simulink model "eovsa_corr_300mhz"  (R2012b)
settings: Solver=VariableStepDiscrete  SolverMode=SingleTasking  StartTime=0.0  StopTime=5000  RelTol=1e-3
undefined symbols (not defined in the file or in its folder): A, B, gcbh, PCIN, sfp, xlBlockLoadCallback, xlipgetpartsetting
libraries: xbsIndex_r4 x5996, casper_library_misc x52, simulink x33, dspsigops x24, xps_library x15, casper_library_delays x2
(part 4 of 65)

== system eovsa_corr_300mhz/auto_shutoff1 ==
  In1 : Inport
  In2 : Inport  Port=2
  In3 : Inport  Port=3
  In4 : Inport  Port=4
  rst : Inport  Port=5
  Accumulator : xbsIndex_r4/Accumulator  operation=Add  n_bits=ceil(log2(clk_freq*1000*acc_time))+bits_in*2  overflow=Wrap  scale=1  rst=on  infoeditControl=reset for floating point data type must be asserted for a minimum of 2 cycles  hasbypass=off  en=off  latency=0  dbl_ovrd=off  msb_inp=100  msb=100  lsb=-100  use_behavioral_HDL=off  implementation=DSP48  block_type=accum
      settings: xl_area=[0, 0, 0, 0, 0, 0, 0]  block_version=10.1.3
  Constant : xbsIndex_r4/Constant  const=2^ceil(log2(clk_freq*1000*acc_time))*max_power  gui_display_data_type=Fixed-point  arith_type=Unsigned  n_bits=ceil(log2(clk_freq*1000*acc_time))+bits_in*2  bin_pt=bin_pt_in*2  preci_type=Single  exp_width=8  frac_width=24  explicit_period=on  period=1  equ=P=C  opselect=C  inp2=PCIN>>17  opr=+  inp1=P  carry=CIN  dbl_ovrd=off  block_type=constant
      settings: block_version=11.4
  Counter1 : xbsIndex_r4/Counter  cnt_type=Free Running  cnt_to=Inf  operation=Up  start_count=0  cnt_by_val=1  arith_type=Unsigned  n_bits=ceil(log2(clk_freq*1000*acc_time))+1  bin_pt=0  load_pin=off  rst=off  en=off  explicit_period=on  period=1  dbl_ovrd=off  use_behavioral_HDL=off  implementation=DSP48  use_rpm=on  block_type=counter
      settings: xl_area=[0, 0, 0, 0, 0, 0, 0]
  Counter2 : xbsIndex_r4/Counter  cnt_type=Free Running  cnt_to=Inf  operation=Up  start_count=0  cnt_by_val=1  arith_type=Unsigned  n_bits=2  bin_pt=0  load_pin=off  rst=off  en=off  explicit_period=on  period=1  dbl_ovrd=off  use_behavioral_HDL=off  implementation=Fabric  block_type=counter
      settings: block_version=11.4
  Delay4 : xbsIndex_r4/Delay  rst=off  infoeditControl=Selection of Reset will increase slice count due to use of real FFs and instead of SRLs  en=off  latency=1  dbl_ovrd=off  reg_retiming=off  block_type=delay
      settings: block_version=11.4
  Logical : xbsIndex_r4/Logical  logical_function=OR  inputs=2  en=off  latency=1  precision=Full  arith_type=Unsigned  n_bits=16  bin_pt=0  align_bp=on  dbl_ovrd=off  block_type=logical
      settings: block_version=11.4
  Mult : xbsIndex_r4/Mult  precision=Full  arith_type="Signed  (2's comp)"  n_bits=8  bin_pt=2  quantization=Truncate  overflow=Wrap  en=off  latency=3  dbl_ovrd=off  use_behavioral_HDL=off  opt=Speed  use_embedded=on  optimum_pipeline=off  pipeline=on  use_rpm=on  placement_style=Rectangular shape  block_type=mult
      settings: xl_area=[0, 0, 0, 0, 0, 0, 0]  block_version=10.1.3
  Mux : xbsIndex_r4/Mux  inputs=4  en=off  latency=1  precision=Full  arith_type="Signed  (2's comp)"  n_bits=8  bin_pt=2  quantization=Truncate  overflow=Wrap  dbl_ovrd=off  block_type=mux
      settings: xl_area=[0, 0, 0, 0, 0, 0, 0]
  Relational : xbsIndex_r4/Relational  mode=a>b  en=off  latency=1  dbl_ovrd=off  block_type=relational
  Slice : xbsIndex_r4/Slice  nbits=1  boolean_output=off  mode=Upper Bit Location + Width  bit1=0  base1=MSB of Input  bit0=0  base0=LSB of Input  dbl_ovrd=off  block_type=slice
      settings: block_version=10.1.3
  Slice1 : xbsIndex_r4/Slice  nbits=1  boolean_output=on  mode=Upper Bit Location + Width  bit1=0  base1=MSB of Input  bit0=0  base0=LSB of Input  dbl_ovrd=off  block_type=slice
  edge_detect : Subsystem  AncestorBlock=casper_library_misc/edge_detect  mask(edge_detect){edge=Both, polarity=Active High, x_in=[0 0.08 0.08 0.16 0.16 0.24 0.24 0.32 0.32 0.4], y_in=[-1 -1  1  1  1  1 -1 -1 -1 -1], x_out=[0.6 0.68 0.68 0.76 0.76 0.84 0.84 0.92 0.92 1], y_out=[-1 -1  1  1 -1 -1  1  1 -1 -1]}
      mask prompts: edge "Edge Type"; polarity "Output Polarity"; x_in "Input X Positions"; y_in "Input Y Positions"; x_out "Output X Positions"; y_out "Output Y Positions"
      mask help: Output is active for one-cycle after each edge of the specified type (i.e. rising, falling or both).
      mask init: same as eovsa_corr_300mhz/edge_detect1
      settings: AttributesFormatString=|
      | both edges
      | active high
      mask Help: Output is active for one-cycle after each edge of the specified type (i.e. rising, falling, or both).  Latency is zero.
      mask TypeOptions edge: Rising | Falling | Both
      mask TypeOptions polarity: Active High | Active Low
      mask Display:
      | plot(x_in_num,0.5+y_in_num*0.2);
      | plot(x_out_num,0.5+y_out_num*0.2);
  en : Outport
  wires:
  Delay4/1 -> Accumulator/1
  Logical/1 -> Accumulator/2
  edge_detect/1(out) -> Slice1/1
  rst/1 -> Logical/2
  Relational/1 -> en/1
  Constant/1 -> Relational/2
  In4/1 -> Mux/5
  In2/1 -> Mux/4
  In3/1 -> Mux/3
  In1/1 -> Mux/2
  Counter2/1 -> Mux/1
  Mux/1 -> Mult/2, Mult/1
  Slice/1 -> edge_detect/1(in)
  Counter1/1 -> Slice/1
  Accumulator/1 -> Relational/1
  Mult/1 -> Delay4/1
  Slice1/1 -> Logical/1

== system eovsa_corr_300mhz/auto_shutoff2 ==
  In1 : Inport
  In2 : Inport  Port=2
  In3 : Inport  Port=3
  In4 : Inport  Port=4
  rst : Inport  Port=5
  Accumulator : xbsIndex_r4/Accumulator  operation=Add  n_bits=ceil(log2(clk_freq*1000*acc_time))+bits_in*2  overflow=Wrap  scale=1  rst=on  infoeditControl=reset for floating point data type must be asserted for a minimum of 2 cycles  hasbypass=off  en=off  latency=0  dbl_ovrd=off  msb_inp=100  msb=100  lsb=-100  use_behavioral_HDL=off  implementation=DSP48  block_type=accum
      settings: xl_area=[0, 0, 0, 0, 0, 0, 0]  block_version=10.1.3
  Constant : xbsIndex_r4/Constant  const=2^ceil(log2(clk_freq*1000*acc_time))*max_power  gui_display_data_type=Fixed-point  arith_type=Unsigned  n_bits=ceil(log2(clk_freq*1000*acc_time))+bits_in*2  bin_pt=bin_pt_in*2  preci_type=Single  exp_width=8  frac_width=24  explicit_period=on  period=1  equ=P=C  opselect=C  inp2=PCIN>>17  opr=+  inp1=P  carry=CIN  dbl_ovrd=off  block_type=constant
      settings: block_version=11.4
  Counter1 : xbsIndex_r4/Counter  cnt_type=Free Running  cnt_to=Inf  operation=Up  start_count=0  cnt_by_val=1  arith_type=Unsigned  n_bits=ceil(log2(clk_freq*1000*acc_time))+1  bin_pt=0  load_pin=off  rst=off  en=off  explicit_period=on  period=1  dbl_ovrd=off  use_behavioral_HDL=off  implementation=DSP48  use_rpm=on  block_type=counter
      settings: xl_area=[0, 0, 0, 0, 0, 0, 0]
  Counter2 : xbsIndex_r4/Counter  cnt_type=Free Running  cnt_to=Inf  operation=Up  start_count=0  cnt_by_val=1  arith_type=Unsigned  n_bits=2  bin_pt=0  load_pin=off  rst=off  en=off  explicit_period=on  period=1  dbl_ovrd=off  use_behavioral_HDL=off  implementation=Fabric  block_type=counter
      settings: block_version=11.4
  Delay4 : xbsIndex_r4/Delay  rst=off  infoeditControl=Selection of Reset will increase slice count due to use of real FFs and instead of SRLs  en=off  latency=1  dbl_ovrd=off  reg_retiming=off  block_type=delay
      settings: block_version=11.4
  Logical : xbsIndex_r4/Logical  logical_function=OR  inputs=2  en=off  latency=1  precision=Full  arith_type=Unsigned  n_bits=16  bin_pt=0  align_bp=on  dbl_ovrd=off  block_type=logical
      settings: block_version=11.4
  Mult : xbsIndex_r4/Mult  precision=Full  arith_type="Signed  (2's comp)"  n_bits=8  bin_pt=2  quantization=Truncate  overflow=Wrap  en=off  latency=3  dbl_ovrd=off  use_behavioral_HDL=off  opt=Speed  use_embedded=on  optimum_pipeline=off  pipeline=on  use_rpm=on  placement_style=Rectangular shape  block_type=mult
      settings: xl_area=[0, 0, 0, 0, 0, 0, 0]  block_version=10.1.3
  Mux : xbsIndex_r4/Mux  inputs=4  en=off  latency=1  precision=Full  arith_type="Signed  (2's comp)"  n_bits=8  bin_pt=2  quantization=Truncate  overflow=Wrap  dbl_ovrd=off  block_type=mux
      settings: xl_area=[0, 0, 0, 0, 0, 0, 0]
  Relational : xbsIndex_r4/Relational  mode=a>b  en=off  latency=1  dbl_ovrd=off  block_type=relational
  Slice : xbsIndex_r4/Slice  nbits=1  boolean_output=off  mode=Upper Bit Location + Width  bit1=0  base1=MSB of Input  bit0=0  base0=LSB of Input  dbl_ovrd=off  block_type=slice
      settings: block_version=10.1.3
  Slice1 : xbsIndex_r4/Slice  nbits=1  boolean_output=on  mode=Upper Bit Location + Width  bit1=0  base1=MSB of Input  bit0=0  base0=LSB of Input  dbl_ovrd=off  block_type=slice
  edge_detect : Subsystem  AncestorBlock=casper_library_misc/edge_detect  mask(edge_detect){edge=Both, polarity=Active High, x_in=[0 0.08 0.08 0.16 0.16 0.24 0.24 0.32 0.32 0.4], y_in=[-1 -1  1  1  1  1 -1 -1 -1 -1], x_out=[0.6 0.68 0.68 0.76 0.76 0.84 0.84 0.92 0.92 1], y_out=[-1 -1  1  1 -1 -1  1  1 -1 -1]}
      mask prompts: edge "Edge Type"; polarity "Output Polarity"; x_in "Input X Positions"; y_in "Input Y Positions"; x_out "Output X Positions"; y_out "Output Y Positions"
      mask help: Output is active for one-cycle after each edge of the specified type (i.e. rising, falling or both).
      mask init: same as eovsa_corr_300mhz/edge_detect1
      settings: AttributesFormatString=|
      | both edges
      | active high
      mask Help: Output is active for one-cycle after each edge of the specified type (i.e. rising, falling, or both).  Latency is zero.
      mask TypeOptions edge: Rising | Falling | Both
      mask TypeOptions polarity: Active High | Active Low
      mask Display:
      | plot(x_in_num,0.5+y_in_num*0.2);
      | plot(x_out_num,0.5+y_out_num*0.2);
  en : Outport
  wires:
  Slice1/1 -> Logical/1
  Mult/1 -> Delay4/1
  Accumulator/1 -> Relational/1
  Counter1/1 -> Slice/1
  Slice/1 -> edge_detect/1(in)
  Mux/1 -> Mult/1, Mult/2
  Counter2/1 -> Mux/1
  In1/1 -> Mux/2
  In3/1 -> Mux/3
  In2/1 -> Mux/4
  In4/1 -> Mux/5
  Constant/1 -> Relational/2
  Relational/1 -> en/1
  rst/1 -> Logical/2
  edge_detect/1(out) -> Slice1/1
  Logical/1 -> Accumulator/2
  Delay4/1 -> Accumulator/1

== system eovsa_corr_300mhz/auto_shutoff3 ==
  In1 : Inport
  In2 : Inport  Port=2
  In3 : Inport  Port=3
  In4 : Inport  Port=4
  rst : Inport  Port=5
  Accumulator : xbsIndex_r4/Accumulator  operation=Add  n_bits=ceil(log2(clk_freq*1000*acc_time))+bits_in*2  overflow=Wrap  scale=1  rst=on  infoeditControl=reset for floating point data type must be asserted for a minimum of 2 cycles  hasbypass=off  en=off  latency=0  dbl_ovrd=off  msb_inp=100  msb=100  lsb=-100  use_behavioral_HDL=off  implementation=DSP48  block_type=accum
      settings: xl_area=[0, 0, 0, 0, 0, 0, 0]  block_version=10.1.3
  Constant : xbsIndex_r4/Constant  const=2^ceil(log2(clk_freq*1000*acc_time))*max_power  gui_display_data_type=Fixed-point  arith_type=Unsigned  n_bits=ceil(log2(clk_freq*1000*acc_time))+bits_in*2  bin_pt=bin_pt_in*2  preci_type=Single  exp_width=8  frac_width=24  explicit_period=on  period=1  equ=P=C  opselect=C  inp2=PCIN>>17  opr=+  inp1=P  carry=CIN  dbl_ovrd=off  block_type=constant
      settings: block_version=11.4
  Counter1 : xbsIndex_r4/Counter  cnt_type=Free Running  cnt_to=Inf  operation=Up  start_count=0  cnt_by_val=1  arith_type=Unsigned  n_bits=ceil(log2(clk_freq*1000*acc_time))+1  bin_pt=0  load_pin=off  rst=off  en=off  explicit_period=on  period=1  dbl_ovrd=off  use_behavioral_HDL=off  implementation=DSP48  use_rpm=on  block_type=counter
      settings: xl_area=[0, 0, 0, 0, 0, 0, 0]
  Counter2 : xbsIndex_r4/Counter  cnt_type=Free Running  cnt_to=Inf  operation=Up  start_count=0  cnt_by_val=1  arith_type=Unsigned  n_bits=2  bin_pt=0  load_pin=off  rst=off  en=off  explicit_period=on  period=1  dbl_ovrd=off  use_behavioral_HDL=off  implementation=Fabric  block_type=counter
      settings: block_version=11.4
  Delay4 : xbsIndex_r4/Delay  rst=off  infoeditControl=Selection of Reset will increase slice count due to use of real FFs and instead of SRLs  en=off  latency=1  dbl_ovrd=off  reg_retiming=off  block_type=delay
      settings: block_version=11.4
  Logical : xbsIndex_r4/Logical  logical_function=OR  inputs=2  en=off  latency=1  precision=Full  arith_type=Unsigned  n_bits=16  bin_pt=0  align_bp=on  dbl_ovrd=off  block_type=logical
      settings: block_version=11.4
  Mult : xbsIndex_r4/Mult  precision=Full  arith_type="Signed  (2's comp)"  n_bits=8  bin_pt=2  quantization=Truncate  overflow=Wrap  en=off  latency=3  dbl_ovrd=off  use_behavioral_HDL=off  opt=Speed  use_embedded=on  optimum_pipeline=off  pipeline=on  use_rpm=on  placement_style=Rectangular shape  block_type=mult
      settings: xl_area=[0, 0, 0, 0, 0, 0, 0]  block_version=10.1.3
  Mux : xbsIndex_r4/Mux  inputs=4  en=off  latency=1  precision=Full  arith_type="Signed  (2's comp)"  n_bits=8  bin_pt=2  quantization=Truncate  overflow=Wrap  dbl_ovrd=off  block_type=mux
      settings: xl_area=[0, 0, 0, 0, 0, 0, 0]
  Relational : xbsIndex_r4/Relational  mode=a>b  en=off  latency=1  dbl_ovrd=off  block_type=relational
  Slice : xbsIndex_r4/Slice  nbits=1  boolean_output=off  mode=Upper Bit Location + Width  bit1=0  base1=MSB of Input  bit0=0  base0=LSB of Input  dbl_ovrd=off  block_type=slice
      settings: block_version=10.1.3
  Slice1 : xbsIndex_r4/Slice  nbits=1  boolean_output=on  mode=Upper Bit Location + Width  bit1=0  base1=MSB of Input  bit0=0  base0=LSB of Input  dbl_ovrd=off  block_type=slice
  edge_detect : Subsystem  AncestorBlock=casper_library_misc/edge_detect  mask(edge_detect){edge=Both, polarity=Active High, x_in=[0 0.08 0.08 0.16 0.16 0.24 0.24 0.32 0.32 0.4], y_in=[-1 -1  1  1  1  1 -1 -1 -1 -1], x_out=[0.6 0.68 0.68 0.76 0.76 0.84 0.84 0.92 0.92 1], y_out=[-1 -1  1  1 -1 -1  1  1 -1 -1]}
      mask prompts: edge "Edge Type"; polarity "Output Polarity"; x_in "Input X Positions"; y_in "Input Y Positions"; x_out "Output X Positions"; y_out "Output Y Positions"
      mask help: Output is active for one-cycle after each edge of the specified type (i.e. rising, falling or both).
      mask init: same as eovsa_corr_300mhz/edge_detect1
      settings: AttributesFormatString=|
      | both edges
      | active high
      mask Help: Output is active for one-cycle after each edge of the specified type (i.e. rising, falling, or both).  Latency is zero.
      mask TypeOptions edge: Rising | Falling | Both
      mask TypeOptions polarity: Active High | Active Low
      mask Display:
      | plot(x_in_num,0.5+y_in_num*0.2);
      | plot(x_out_num,0.5+y_out_num*0.2);
  en : Outport
  wires:
  Delay4/1 -> Accumulator/1
  Logical/1 -> Accumulator/2
  edge_detect/1(out) -> Slice1/1
  rst/1 -> Logical/2
  Relational/1 -> en/1
  Constant/1 -> Relational/2
  In4/1 -> Mux/5
  In2/1 -> Mux/4
  In3/1 -> Mux/3
  In1/1 -> Mux/2
  Counter2/1 -> Mux/1
  Mux/1 -> Mult/2, Mult/1
  Slice/1 -> edge_detect/1(in)
  Counter1/1 -> Slice/1
  Accumulator/1 -> Relational/1
  Mult/1 -> Delay4/1
  Slice1/1 -> Logical/1

== system eovsa_corr_300mhz/bus_create ==
  in1 : Inport
  in2 : Inport  Port=2
  in3 : Inport  Port=3
  in4 : Inport  Port=4
  in5 : Inport  Port=5
  in6 : Inport  Port=6
  in7 : Inport  Port=7
  in8 : Inport  Port=8
  concatenate : xbsIndex_r4/Concat  num_inputs=8  dbl_ovrd=off  block_type=concat
  reinterpret{1..8} (8 alike) : xbsIndex_r4/Reinterpret  force_arith_type=on  arith_type=Unsigned  force_bin_pt=on  bin_pt=0  block_type=reinterpret
      reinterpret1 settings: infoedit="Changes signal type without altering the binary representation.   You can changed the signal between signed and unsigned, and relocate the binary point.<br><br>Hardware notes: In hardware this block costs nothing.<br><br>Example:  Suppose the input is 6 bits wide, signed, with 2 fractional bits, and the output is forced to unsigned with 0 fractional bits.  Then an input of -2.0 (1110.00 in binary 2's complement) becomes an output of 56 (111000 in binary)."
      reinterpret2 settings: infoedit="Changes signal type without altering the binary representation.   You can changed the signal between signed and unsigned, and relocate the binary point.<br><br>Hardware notes: In hardware this block costs nothing.<br><br>Example:  Suppose the input is 6 bits wide, signed, with 2 fractional bits, and the output is forced to unsigned with 0 fractional bits.  Then an input of -2.0 (1110.00 in binary 2's complement) becomes an output of 56 (111000 in binary)."
  bus_out : Outport
  wires:
  concatenate/1 -> bus_out/1
  in1/1 -> reinterpret1/1
  reinterpret1/1 -> concatenate/1
  in2/1 -> reinterpret2/1
  reinterpret2/1 -> concatenate/2
  in3/1 -> reinterpret3/1
  reinterpret3/1 -> concatenate/3
  in4/1 -> reinterpret4/1
  reinterpret4/1 -> concatenate/4
  in5/1 -> reinterpret5/1
  reinterpret5/1 -> concatenate/5
  in6/1 -> reinterpret6/1
  reinterpret6/1 -> concatenate/6
  in7/1 -> reinterpret7/1
  reinterpret7/1 -> concatenate/7
  in8/1 -> reinterpret8/1
  reinterpret8/1 -> concatenate/8

== system eovsa_corr_300mhz/bus_expand7 ==
  bus_in : Inport
  reinterpret{1..4} (4 alike) : xbsIndex_r4/Reinterpret  force_arith_type=on  arith_type=Unsigned  force_bin_pt=on  bin_pt=0  block_type=reinterpret
  slice1 : xbsIndex_r4/Slice  nbits=32  boolean_output=off  mode=Upper Bit Location + Width  bit1=-96  base1=MSB of Input  bit0=0  base0=LSB of Input  dbl_ovrd=off  block_type=slice
  slice2 : xbsIndex_r4/Slice  nbits=32  boolean_output=off  mode=Upper Bit Location + Width  bit1=-64  base1=MSB of Input  bit0=0  base0=LSB of Input  dbl_ovrd=off  block_type=slice
  slice3 : xbsIndex_r4/Slice  nbits=32  boolean_output=off  mode=Upper Bit Location + Width  bit1=-32  base1=MSB of Input  bit0=0  base0=LSB of Input  dbl_ovrd=off  block_type=slice
  slice4 : xbsIndex_r4/Slice  nbits=32  boolean_output=off  mode=Upper Bit Location + Width  bit1=0  base1=MSB of Input  bit0=0  base0=LSB of Input  dbl_ovrd=off  block_type=slice
  msb_out4 : Outport
  out3 : Outport  Port=2
  out2 : Outport  Port=3
  lsb_out1 : Outport  Port=4
  wires:
  bus_in/1 -> slice4/1, slice3/1, slice2/1, slice1/1
  slice4/1 -> reinterpret4/1
  reinterpret4/1 -> msb_out4/1
  slice3/1 -> reinterpret3/1
  reinterpret3/1 -> out3/1
  slice2/1 -> reinterpret2/1
  reinterpret2/1 -> out2/1
  slice1/1 -> reinterpret1/1
  reinterpret1/1 -> lsb_out1/1

== system eovsa_corr_300mhz/coarse_delay ==
  sync : Inport
  new_acc : Inport  Port=2
  delay00 : Inport  Port=3
  adc0_pol0 : Inport  Port=4
  delay01 : Inport  Port=5
  adc0_pol1 : Inport  Port=6
  delay10 : Inport  Port=7
  adc1_pol0 : Inport  Port=8
  delay11 : Inport  Port=9
  adc1_pol1 : Inport  Port=10
  bus_create : Subsystem  AncestorBlock=casper_library_flow_control/bus_create  mask(bus_create){inputNum=4}
      mask prompts: inputNum "Number of inputs:"
      mask init:
      | bus_create_init(gcb,...
      |     'inputNum', inputNum);
  bus_create1 : Subsystem  AncestorBlock=casper_library_flow_control/bus_create  mask(bus_create){inputNum=4}
      mask prompts: inputNum "Number of inputs:"
      mask init:
      | bus_create_init(gcb,...
      |     'inputNum', inputNum);
  bus_create2 : Subsystem  AncestorBlock=casper_library_flow_control/bus_create  mask(bus_create){inputNum=4}
      mask prompts: inputNum "Number of inputs:"
      mask init:
      | bus_create_init(gcb,...
      |     'inputNum', inputNum);
  bus_create3 : Subsystem  AncestorBlock=casper_library_flow_control/bus_create  mask(bus_create){inputNum=4}
      mask prompts: inputNum "Number of inputs:"
      mask init:
      | bus_create_init(gcb,...
      |     'inputNum', inputNum);
  bus_expand : Subsystem  AncestorBlock=casper_library_flow_control/bus_expand  mask(bus_expand){mode=divisions of equal size, outputNum=4, outputWidth=8, outputBinaryPt=7, outputArithmeticType=1, show_format=off, outputToWorkspace=off, variablePrefix=out, outputToModelAsWell=on}
      mask prompts: outputNum "Number of outputs:"; outputWidth "Output width:"; outputBinaryPt "Output binary point position:"; outputArithmeticType "Output arithmetic type (ufix=0, fix=1, bool=2):"; show_format "Print format string?"; outputToWorkspace "Output to workspace?"; variablePrefix "Variable name prefix:"; outputToModelAsWell "Output to model as well?"
      mask help:
      | Expands a 'bus' made using a bus_create or Xilinx
      | concat block.
      | The input will be divided into the specified number
      | of outputs with the specified arithmetic types.
      | Divisions are made from most significant bit.
      mask init: same as eovsa_corr_300mhz/bus_expand7
      settings: AttributesFormatString=4 outputs
      mask TypeOptions mode: divisions of equal size | divisions of arbitrary size
      mask Callback mode: bus_expand_callback();
      mask Callback outputWidth: bus_expand_callback();
      mask Callback outputToWorkspace: bus_expand_callback();
  bus_expand1 : Subsystem  AncestorBlock=casper_library_flow_control/bus_expand  mask(bus_expand){mode=divisions of equal size, outputNum=4, outputWidth=8, outputBinaryPt=7, outputArithmeticType=1, show_format=off, outputToWorkspace=off, variablePrefix=out, outputToModelAsWell=on}
      mask prompts: outputNum "Number of outputs:"; outputWidth "Output width:"; outputBinaryPt "Output binary point position:"; outputArithmeticType "Output arithmetic type (ufix=0, fix=1, bool=2):"; show_format "Print format string?"; outputToWorkspace "Output to workspace?"; variablePrefix "Variable name prefix:"; outputToModelAsWell "Output to model as well?"
      mask help:
      | Expands a 'bus' made using a bus_create or Xilinx
      | concat block.
      | The input will be divided into the specified number
      | of outputs with the specified arithmetic types.
      | Divisions are made from most significant bit.
      mask init: same as eovsa_corr_300mhz/bus_expand7
      settings: AttributesFormatString=4 outputs
      mask TypeOptions mode: divisions of equal size | divisions of arbitrary size
      mask Callback mode: bus_expand_callback();
      mask Callback outputWidth: bus_expand_callback();
      mask Callback outputToWorkspace: bus_expand_callback();
  bus_expand2 : Subsystem  AncestorBlock=casper_library_flow_control/bus_expand  mask(bus_expand){mode=divisions of equal size, outputNum=4, outputWidth=8, outputBinaryPt=7, outputArithmeticType=1, show_format=off, outputToWorkspace=off, variablePrefix=out, outputToModelAsWell=on}
      mask prompts: outputNum "Number of outputs:"; outputWidth "Output width:"; outputBinaryPt "Output binary point position:"; outputArithmeticType "Output arithmetic type (ufix=0, fix=1, bool=2):"; show_format "Print format string?"; outputToWorkspace "Output to workspace?"; variablePrefix "Variable name prefix:"; outputToModelAsWell "Output to model as well?"
      mask help:
      | Expands a 'bus' made using a bus_create or Xilinx
      | concat block.
      | The input will be divided into the specified number
      | of outputs with the specified arithmetic types.
      | Divisions are made from most significant bit.
      mask init: same as eovsa_corr_300mhz/bus_expand7
      settings: AttributesFormatString=4 outputs
      mask TypeOptions mode: divisions of equal size | divisions of arbitrary size
      mask Callback mode: bus_expand_callback();
      mask Callback outputWidth: bus_expand_callback();
      mask Callback outputToWorkspace: bus_expand_callback();
  bus_expand3 : Subsystem  AncestorBlock=casper_library_flow_control/bus_expand  mask(bus_expand){mode=divisions of equal size, outputNum=4, outputWidth=8, outputBinaryPt=7, outputArithmeticType=1, show_format=off, outputToWorkspace=off, variablePrefix=out, outputToModelAsWell=on}
      mask prompts: outputNum "Number of outputs:"; outputWidth "Output width:"; outputBinaryPt "Output binary point position:"; outputArithmeticType "Output arithmetic type (ufix=0, fix=1, bool=2):"; show_format "Print format string?"; outputToWorkspace "Output to workspace?"; variablePrefix "Variable name prefix:"; outputToModelAsWell "Output to model as well?"
      mask help:
      | Expands a 'bus' made using a bus_create or Xilinx
      | concat block.
      | The input will be divided into the specified number
      | of outputs with the specified arithmetic types.
      | Divisions are made from most significant bit.
      mask init: same as eovsa_corr_300mhz/bus_expand7
      settings: AttributesFormatString=4 outputs
      mask TypeOptions mode: divisions of equal size | divisions of arbitrary size
      mask Callback mode: bus_expand_callback();
      mask Callback outputWidth: bus_expand_callback();
      mask Callback outputToWorkspace: bus_expand_callback();
  coarse_delay00 : xbsIndex_r4/Black Box  init_code=coarse_delay_core_config  sim_method=Inactive  verbose=off  block_type=blackbox2
      settings: block_version=11.4
  coarse_delay01 : xbsIndex_r4/Black Box  init_code=coarse_delay_core_config  sim_method=Inactive  verbose=off  block_type=blackbox2
      settings: block_version=11.4
  coarse_delay10 : xbsIndex_r4/Black Box  init_code=coarse_delay_core_config  sim_method=Inactive  verbose=off  block_type=blackbox2
      settings: block_version=11.4
  coarse_delay11 : xbsIndex_r4/Black Box  init_code=coarse_delay_core_config  sim_method=Inactive  verbose=off  block_type=blackbox2
      settings: block_version=11.4
  sync00 : Outport
  adc0_pol0_out : Outport  Port=2
  adc0_pol1_out : Outport  Port=3
  adc1_pol0_out : Outport  Port=4
  adc1_pol1_out : Outport  Port=5
  wires:
  delay00/1 -> coarse_delay00/2
  coarse_delay00/1 -> sync00/1
  sync/1 -> [sync_coarse_delay]
  new_acc/1 -> [new_acc_coarse_delay]
  [sync_coarse_delay] -> coarse_delay00/1
  bus_create/1(bus_out) -> adc0_pol0_out/1
  adc0_pol0/1 -> bus_expand/1(bus_in)
  coarse_delay00/2 -> bus_create/1(in1)
  coarse_delay00/3 -> bus_create/2(in2)
  coarse_delay00/4 -> bus_create/3(in3)
  coarse_delay00/5 -> bus_create/4(in4)
  bus_expand/1(msb_out4) -> coarse_delay00/4
  bus_expand/2(out3) -> coarse_delay00/5
  bus_expand/3(out2) -> coarse_delay00/6
  bus_expand/4(lsb_out1) -> coarse_delay00/7
  [new_acc_coarse_delay] -> coarse_delay00/3
  [sync_coarse_delay] -> coarse_delay01/1
  coarse_delay01/2 -> bus_create1/1(in1)
  coarse_delay01/3 -> bus_create1/2(in2)
  coarse_delay01/4 -> bus_create1/3(in3)
  coarse_delay01/5 -> bus_create1/4(in4)
  bus_expand1/1(msb_out4) -> coarse_delay01/4
  bus_expand1/2(out3) -> coarse_delay01/5
  bus_expand1/3(out2) -> coarse_delay01/6
  bus_expand1/4(lsb_out1) -> coarse_delay01/7
  [new_acc_coarse_delay] -> coarse_delay01/3
  bus_create1/1(bus_out) -> adc0_pol1_out/1
  [sync_coarse_delay] -> coarse_delay10/1
  coarse_delay10/2 -> bus_create2/1(in1)
  coarse_delay10/3 -> bus_create2/2(in2)
  coarse_delay10/4 -> bus_create2/3(in3)
  coarse_delay10/5 -> bus_create2/4(in4)
  bus_expand2/1(msb_out4) -> coarse_delay10/4
  bus_expand2/2(out3) -> coarse_delay10/5
  bus_expand2/3(out2) -> coarse_delay10/6
  bus_expand2/4(lsb_out1) -> coarse_delay10/7
  [new_acc_coarse_delay] -> coarse_delay10/3
  bus_create2/1(bus_out) -> adc1_pol0_out/1
  [sync_coarse_delay] -> coarse_delay11/1
  coarse_delay11/2 -> bus_create3/1(in1)
  coarse_delay11/3 -> bus_create3/2(in2)
  coarse_delay11/4 -> bus_create3/3(in3)
  coarse_delay11/5 -> bus_create3/4(in4)
  bus_expand3/1(msb_out4) -> coarse_delay11/4
  bus_expand3/2(out3) -> coarse_delay11/5
  bus_expand3/3(out2) -> coarse_delay11/6
  bus_expand3/4(lsb_out1) -> coarse_delay11/7
  [new_acc_coarse_delay] -> coarse_delay11/3
  bus_create3/1(bus_out) -> adc1_pol1_out/1
  delay01/1 -> coarse_delay01/2
  adc0_pol1/1 -> bus_expand1/1(bus_in)
  delay10/1 -> coarse_delay10/2
  adc1_pol0/1 -> bus_expand2/1(bus_in)
  delay11/1 -> coarse_delay11/2
  adc1_pol1/1 -> bus_expand3/1(bus_in)

== system eovsa_corr_300mhz/decat1 ==
  i1 : Inport
  Reinterpret{1..4} (4 alike) : xbsIndex_r4/Reinterpret  force_arith_type=on  arith_type="Signed  (2's comp)"  force_bin_pt=on  bin_pt=7  block_type=reinterpret
      settings: infoedit="Changes signal type without altering the binary representation.   You can changed the signal between signed and unsigned, and relocate the binary point.<br><br>Hardware notes: In hardware this block costs nothing.<br><br>Example:  Suppose the input is 6 bits wide, signed, with 2 fractional bits, and the output is forced to unsigned with 0 fractional bits.  Then an input of -2.0 (1110.00 in binary 2's complement) becomes an output of 56 (111000 in binary)."  block_version=10.1.3
  Slice15 : xbsIndex_r4/Slice  nbits=8  boolean_output=off  mode=Lower Bit Location + Width  bit1=0  base1=MSB of Input  bit0=8  base0=LSB of Input  dbl_ovrd=off  block_type=slice
      settings: infoedit="Extracts a given range of bits from each input sample and presents it at the output.  The output type is ordinarily unsigned with binary point at zero, but can be Boolean when the slice is one bit wide.<P><P>Hardware notes: In hardware this block costs nothing."  block_version=10.1.3
  Slice16 : xbsIndex_r4/Slice  nbits=8  boolean_output=off  mode=Lower Bit Location + Width  bit1=0  base1=MSB of Input  bit0=16  base0=LSB of Input  dbl_ovrd=off  block_type=slice
      settings: infoedit="Extracts a given range of bits from each input sample and presents it at the output.  The output type is ordinarily unsigned with binary point at zero, but can be Boolean when the slice is one bit wide.<P><P>Hardware notes: In hardware this block costs nothing."  block_version=10.1.3
  Slice17 : xbsIndex_r4/Slice  nbits=8  boolean_output=off  mode=Lower Bit Location + Width  bit1=0  base1=MSB of Input  bit0=24  base0=LSB of Input  dbl_ovrd=off  block_type=slice
      settings: infoedit="Extracts a given range of bits from each input sample and presents it at the output.  The output type is ordinarily unsigned with binary point at zero, but can be Boolean when the slice is one bit wide.<P><P>Hardware notes: In hardware this block costs nothing."  block_version=10.1.3
  Slice9 : xbsIndex_r4/Slice  nbits=8  boolean_output=off  mode=Lower Bit Location + Width  bit1=0  base1=MSB of Input  bit0=0  base0=LSB of Input  dbl_ovrd=off  block_type=slice
      settings: infoedit="Extracts a given range of bits from each input sample and presents it at the output.  The output type is ordinarily unsigned with binary point at zero, but can be Boolean when the slice is one bit wide.<P><P>Hardware notes: In hardware this block costs nothing."  block_version=10.1.3
  o1 : Outport
  o2 : Outport  Port=2
  o3 : Outport  Port=3
  o4 : Outport  Port=4
  wires:
  i1/1 -> Slice17/1, Slice16/1, Slice9/1, Slice15/1
  Slice17/1 -> Reinterpret2/1
  Slice16/1 -> Reinterpret1/1
  Slice15/1 -> Reinterpret3/1
  Slice9/1 -> Reinterpret4/1
  Reinterpret2/1 -> o1/1
  Reinterpret1/1 -> o2/1
  Reinterpret3/1 -> o3/1
  Reinterpret4/1 -> o4/1

== system eovsa_corr_300mhz/decat2 ==
  i1 : Inport
  Reinterpret{1..4} (4 alike) : xbsIndex_r4/Reinterpret  force_arith_type=on  arith_type="Signed  (2's comp)"  force_bin_pt=on  bin_pt=7  block_type=reinterpret
      settings: infoedit="Changes signal type without altering the binary representation.   You can changed the signal between signed and unsigned, and relocate the binary point.<br><br>Hardware notes: In hardware this block costs nothing.<br><br>Example:  Suppose the input is 6 bits wide, signed, with 2 fractional bits, and the output is forced to unsigned with 0 fractional bits.  Then an input of -2.0 (1110.00 in binary 2's complement) becomes an output of 56 (111000 in binary)."  block_version=10.1.3
  Slice15 : xbsIndex_r4/Slice  nbits=8  boolean_output=off  mode=Lower Bit Location + Width  bit1=0  base1=MSB of Input  bit0=8  base0=LSB of Input  dbl_ovrd=off  block_type=slice
      settings: infoedit="Extracts a given range of bits from each input sample and presents it at the output.  The output type is ordinarily unsigned with binary point at zero, but can be Boolean when the slice is one bit wide.<P><P>Hardware notes: In hardware this block costs nothing."  block_version=10.1.3
  Slice16 : xbsIndex_r4/Slice  nbits=8  boolean_output=off  mode=Lower Bit Location + Width  bit1=0  base1=MSB of Input  bit0=16  base0=LSB of Input  dbl_ovrd=off  block_type=slice
      settings: infoedit="Extracts a given range of bits from each input sample and presents it at the output.  The output type is ordinarily unsigned with binary point at zero, but can be Boolean when the slice is one bit wide.<P><P>Hardware notes: In hardware this block costs nothing."  block_version=10.1.3
  Slice17 : xbsIndex_r4/Slice  nbits=8  boolean_output=off  mode=Lower Bit Location + Width  bit1=0  base1=MSB of Input  bit0=24  base0=LSB of Input  dbl_ovrd=off  block_type=slice
      settings: infoedit="Extracts a given range of bits from each input sample and presents it at the output.  The output type is ordinarily unsigned with binary point at zero, but can be Boolean when the slice is one bit wide.<P><P>Hardware notes: In hardware this block costs nothing."  block_version=10.1.3
  Slice9 : xbsIndex_r4/Slice  nbits=8  boolean_output=off  mode=Lower Bit Location + Width  bit1=0  base1=MSB of Input  bit0=0  base0=LSB of Input  dbl_ovrd=off  block_type=slice
      settings: infoedit="Extracts a given range of bits from each input sample and presents it at the output.  The output type is ordinarily unsigned with binary point at zero, but can be Boolean when the slice is one bit wide.<P><P>Hardware notes: In hardware this block costs nothing."  block_version=10.1.3
  o1 : Outport
  o2 : Outport  Port=2
  o3 : Outport  Port=3
  o4 : Outport  Port=4
  wires:
  Reinterpret4/1 -> o4/1
  Reinterpret3/1 -> o3/1
  Reinterpret1/1 -> o2/1
  Reinterpret2/1 -> o1/1
  Slice9/1 -> Reinterpret4/1
  Slice15/1 -> Reinterpret3/1
  Slice16/1 -> Reinterpret1/1
  Slice17/1 -> Reinterpret2/1
  i1/1 -> Slice15/1, Slice9/1, Slice16/1, Slice17/1

== system eovsa_corr_300mhz/decat3 ==
  i1 : Inport
  Reinterpret{1..4} (4 alike) : xbsIndex_r4/Reinterpret  force_arith_type=on  arith_type="Signed  (2's comp)"  force_bin_pt=on  bin_pt=7  block_type=reinterpret
      settings: infoedit="Changes signal type without altering the binary representation.   You can changed the signal between signed and unsigned, and relocate the binary point.<br><br>Hardware notes: In hardware this block costs nothing.<br><br>Example:  Suppose the input is 6 bits wide, signed, with 2 fractional bits, and the output is forced to unsigned with 0 fractional bits.  Then an input of -2.0 (1110.00 in binary 2's complement) becomes an output of 56 (111000 in binary)."  block_version=10.1.3
  Slice15 : xbsIndex_r4/Slice  nbits=8  boolean_output=off  mode=Lower Bit Location + Width  bit1=0  base1=MSB of Input  bit0=8  base0=LSB of Input  dbl_ovrd=off  block_type=slice
      settings: infoedit="Extracts a given range of bits from each input sample and presents it at the output.  The output type is ordinarily unsigned with binary point at zero, but can be Boolean when the slice is one bit wide.<P><P>Hardware notes: In hardware this block costs nothing."  block_version=10.1.3
  Slice16 : xbsIndex_r4/Slice  nbits=8  boolean_output=off  mode=Lower Bit Location + Width  bit1=0  base1=MSB of Input  bit0=16  base0=LSB of Input  dbl_ovrd=off  block_type=slice
      settings: infoedit="Extracts a given range of bits from each input sample and presents it at the output.  The output type is ordinarily unsigned with binary point at zero, but can be Boolean when the slice is one bit wide.<P><P>Hardware notes: In hardware this block costs nothing."  block_version=10.1.3
  Slice17 : xbsIndex_r4/Slice  nbits=8  boolean_output=off  mode=Lower Bit Location + Width  bit1=0  base1=MSB of Input  bit0=24  base0=LSB of Input  dbl_ovrd=off  block_type=slice
      settings: infoedit="Extracts a given range of bits from each input sample and presents it at the output.  The output type is ordinarily unsigned with binary point at zero, but can be Boolean when the slice is one bit wide.<P><P>Hardware notes: In hardware this block costs nothing."  block_version=10.1.3
  Slice9 : xbsIndex_r4/Slice  nbits=8  boolean_output=off  mode=Lower Bit Location + Width  bit1=0  base1=MSB of Input  bit0=0  base0=LSB of Input  dbl_ovrd=off  block_type=slice
      settings: infoedit="Extracts a given range of bits from each input sample and presents it at the output.  The output type is ordinarily unsigned with binary point at zero, but can be Boolean when the slice is one bit wide.<P><P>Hardware notes: In hardware this block costs nothing."  block_version=10.1.3
  o1 : Outport
  o2 : Outport  Port=2
  o3 : Outport  Port=3
  o4 : Outport  Port=4
  wires:
  Reinterpret4/1 -> o4/1
  Reinterpret3/1 -> o3/1
  Reinterpret1/1 -> o2/1
  Reinterpret2/1 -> o1/1
  Slice9/1 -> Reinterpret4/1
  Slice15/1 -> Reinterpret3/1
  Slice16/1 -> Reinterpret1/1
  Slice17/1 -> Reinterpret2/1
  i1/1 -> Slice15/1, Slice9/1, Slice16/1, Slice17/1

== system eovsa_corr_300mhz/decat4 ==
  i1 : Inport
  Reinterpret{1..4} (4 alike) : xbsIndex_r4/Reinterpret  force_arith_type=on  arith_type="Signed  (2's comp)"  force_bin_pt=on  bin_pt=7  block_type=reinterpret
      settings: infoedit="Changes signal type without altering the binary representation.   You can changed the signal between signed and unsigned, and relocate the binary point.<br><br>Hardware notes: In hardware this block costs nothing.<br><br>Example:  Suppose the input is 6 bits wide, signed, with 2 fractional bits, and the output is forced to unsigned with 0 fractional bits.  Then an input of -2.0 (1110.00 in binary 2's complement) becomes an output of 56 (111000 in binary)."  block_version=10.1.3
  Slice15 : xbsIndex_r4/Slice  nbits=8  boolean_output=off  mode=Lower Bit Location + Width  bit1=0  base1=MSB of Input  bit0=8  base0=LSB of Input  dbl_ovrd=off  block_type=slice
      settings: infoedit="Extracts a given range of bits from each input sample and presents it at the output.  The output type is ordinarily unsigned with binary point at zero, but can be Boolean when the slice is one bit wide.<P><P>Hardware notes: In hardware this block costs nothing."  block_version=10.1.3
  Slice16 : xbsIndex_r4/Slice  nbits=8  boolean_output=off  mode=Lower Bit Location + Width  bit1=0  base1=MSB of Input  bit0=16  base0=LSB of Input  dbl_ovrd=off  block_type=slice
      settings: infoedit="Extracts a given range of bits from each input sample and presents it at the output.  The output type is ordinarily unsigned with binary point at zero, but can be Boolean when the slice is one bit wide.<P><P>Hardware notes: In hardware this block costs nothing."  block_version=10.1.3
  Slice17 : xbsIndex_r4/Slice  nbits=8  boolean_output=off  mode=Lower Bit Location + Width  bit1=0  base1=MSB of Input  bit0=24  base0=LSB of Input  dbl_ovrd=off  block_type=slice
      settings: infoedit="Extracts a given range of bits from each input sample and presents it at the output.  The output type is ordinarily unsigned with binary point at zero, but can be Boolean when the slice is one bit wide.<P><P>Hardware notes: In hardware this block costs nothing."  block_version=10.1.3
  Slice9 : xbsIndex_r4/Slice  nbits=8  boolean_output=off  mode=Lower Bit Location + Width  bit1=0  base1=MSB of Input  bit0=0  base0=LSB of Input  dbl_ovrd=off  block_type=slice
      settings: infoedit="Extracts a given range of bits from each input sample and presents it at the output.  The output type is ordinarily unsigned with binary point at zero, but can be Boolean when the slice is one bit wide.<P><P>Hardware notes: In hardware this block costs nothing."  block_version=10.1.3
  o1 : Outport
  o2 : Outport  Port=2
  o3 : Outport  Port=3
  o4 : Outport  Port=4
  wires:
  i1/1 -> Slice17/1, Slice16/1, Slice9/1, Slice15/1
  Slice17/1 -> Reinterpret2/1
  Slice16/1 -> Reinterpret1/1
  Slice15/1 -> Reinterpret3/1
  Slice9/1 -> Reinterpret4/1
  Reinterpret2/1 -> o1/1
  Reinterpret1/1 -> o2/1
  Reinterpret3/1 -> o3/1
  Reinterpret4/1 -> o4/1

== system eovsa_corr_300mhz/edge_detect1 ==
  in : Inport
  Delay : xbsIndex_r4/Delay  rst=off  infoeditControl=Selection of Reset will increase slice count due to use of real FFs and instead of SRLs  en=off  latency=1  dbl_ovrd=off  reg_retiming=on  block_type=delay
      settings: xl_area=[0, 0, 0, 0, 0, 0, 0]
  Inverter : xbsIndex_r4/Inverter  en=off  latency=0  dbl_ovrd=off  block_type=inv
      settings: xl_area=[0, 0, 0, 0, 0, 0, 0]
  edge_op : xbsIndex_r4/Logical  logical_function=NOR  inputs=2  en=off  latency=0  precision=Full  arith_type=Unsigned  n_bits=8  bin_pt=2  align_bp=on  dbl_ovrd=off  block_type=logical
      settings: xl_area=[0, 0, 0, 0, 0, 0, 0]
  out : Outport
  wires:
  Inverter/1 -> edge_op/1
  edge_op/1 -> out/1
  in/1 -> Inverter/1, Delay/1
  Delay/1 -> edge_op/2

== system eovsa_corr_300mhz/edge_detect12 ==
  in : Inport
  Delay : xbsIndex_r4/Delay  rst=off  infoeditControl=Selection of Reset will increase slice count due to use of real FFs and instead of SRLs  en=off  latency=1  dbl_ovrd=off  reg_retiming=on  block_type=delay
      settings: xl_area=[0, 0, 0, 0, 0, 0, 0]
  Inverter : xbsIndex_r4/Inverter  en=off  latency=0  dbl_ovrd=off  block_type=inv
      settings: xl_area=[0, 0, 0, 0, 0, 0, 0]
  edge_op : xbsIndex_r4/Logical  logical_function=NOR  inputs=2  en=off  latency=0  precision=Full  arith_type=Unsigned  n_bits=8  bin_pt=2  align_bp=on  dbl_ovrd=off  block_type=logical
      settings: xl_area=[0, 0, 0, 0, 0, 0, 0]
  out : Outport
  wires:
  Inverter/1 -> edge_op/1
  edge_op/1 -> out/1
  in/1 -> Inverter/1, Delay/1
  Delay/1 -> edge_op/2

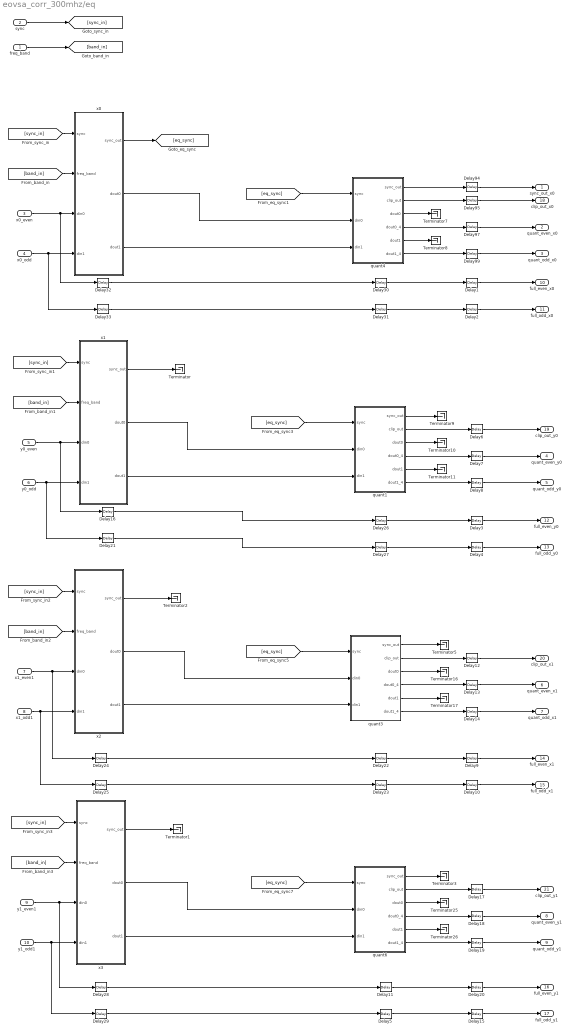
== system eovsa_corr_300mhz/eq ==
  freq_band : Inport
  sync : Inport  Port=2
  x0_even : Inport  Port=3
  x0_odd : Inport  Port=4
  y0_even : Inport  Port=5
  y0_odd : Inport  Port=6
  x1_even1 : Inport  Port=7
  x1_odd1 : Inport  Port=8
  y1_even1 : Inport  Port=9
  y1_odd1 : Inport  Port=10
  Delay{1..4,6..10,12..13,15,17..20,95,97,99} (19 alike) : xbsIndex_r4/Delay  rst=off  infoeditControl=Selection of Reset will increase slice count due to use of real FFs and instead of SRLs  en=off  latency=1  dbl_ovrd=off  reg_retiming=on  block_type=delay
      settings: block_version=11.4
  Delay{5,11,22..23,26..27,30..31} (8 alike) : xbsIndex_r4/Delay  rst=off  infoeditControl=Selection of Reset will increase slice count due to use of real FFs and instead of SRLs  en=off  latency=6  dbl_ovrd=off  reg_retiming=on  block_type=delay
      settings: block_version=11.4
  Delay14 : xbsIndex_r4/Delay  rst=off  infoeditControl=Selection of Reset will increase slice count due to use of real FFs and instead of SRLs  en=off  latency=1  dbl_ovrd=off  reg_retiming=off  block_type=delay
      settings: block_version=11.4
  Delay{16,21,24..25,28..29,32..33} (8 alike) : xbsIndex_r4/Delay  rst=off  infoeditControl=Selection of Reset will increase slice count due to use of real FFs and instead of SRLs  en=off  latency=9  dbl_ovrd=off  reg_retiming=on  block_type=delay
      settings: block_version=11.4
  Delay94 : xbsIndex_r4/Delay  rst=off  infoeditControl=Selection of Reset will increase slice count due to use of real FFs and instead of SRLs  en=off  latency=1  dbl_ovrd=off  reg_retiming=off  block_type=delay
      settings: block_version=11.4
  Terminator{,1..3,5,7..11,16..17,25..26} (14 alike) : Terminator
  quant1 : Subsystem  mask{pol_n_bits=pol_n_bits + 16 + 1, pol_bin_pt=pol_bin_pt + coeff_bin_pt, pol_op_bits=pol_op_bits, pol_op_bin_pt=pol_op_bin_pt}
      mask prompts: pol_n_bits "Number of bits in"; pol_bin_pt "Binary point in"; pol_op_bits "Number of bits out"; pol_op_bin_pt "Binary point out"
  quant3 : Subsystem  mask{pol_n_bits=pol_n_bits + 16 + 1, pol_bin_pt=pol_bin_pt + coeff_bin_pt, pol_op_bits=pol_op_bits, pol_op_bin_pt=pol_op_bin_pt}
      mask prompts: pol_n_bits "Number of bits in"; pol_bin_pt "Binary point in"; pol_op_bits "Number of bits out"; pol_op_bin_pt "Binary point out"
  quant4 : Subsystem  mask{pol_n_bits=pol_n_bits + 16 + 1, pol_bin_pt=pol_bin_pt + coeff_bin_pt, pol_op_bits=pol_op_bits, pol_op_bin_pt=pol_op_bin_pt}
      mask prompts: pol_n_bits "Number of bits in"; pol_bin_pt "Binary point in"; pol_op_bits "Number of bits out"; pol_op_bin_pt "Binary point out"
  quant6 : Subsystem  mask{pol_n_bits=pol_n_bits + 16 + 1, pol_bin_pt=pol_bin_pt + coeff_bin_pt, pol_op_bits=pol_op_bits, pol_op_bin_pt=pol_op_bin_pt}
      mask prompts: pol_n_bits "Number of bits in"; pol_bin_pt "Binary point in"; pol_op_bits "Number of bits out"; pol_op_bin_pt "Binary point out"
  x0 : Subsystem
  x1 : Subsystem
  x2 : Subsystem
  x3 : Subsystem
  sync_out_x0 : Outport
  quant_even_x0 : Outport  Port=2
  quant_odd_x0 : Outport  Port=3
  quant_even_y0 : Outport  Port=4
  quant_odd_y0 : Outport  Port=5
  quant_even_x1 : Outport  Port=6
  quant_odd_x1 : Outport  Port=7
  quant_even_y1 : Outport  Port=8
  quant_odd_y1 : Outport  Port=9
  full_even_x0 : Outport  Port=10
  full_odd_x0 : Outport  Port=11
  full_even_y0 : Outport  Port=12
  full_odd_y0 : Outport  Port=13
  full_even_x1 : Outport  Port=14
  full_odd_x1 : Outport  Port=15
  full_even_y1 : Outport  Port=16
  full_odd_y1 : Outport  Port=17
  clip_out_x0 : Outport  Port=18
  clip_out_y0 : Outport  Port=19
  clip_out_x1 : Outport  Port=20
  clip_out_y1 : Outport  Port=21
  wires:
  Delay99/1 -> quant_odd_x0/1
  Delay97/1 -> quant_even_x0/1
  Delay95/1 -> clip_out_x0/1
  Delay94/1 -> sync_out_x0/1
  quant4/6(dout1_4) -> Delay99/1
  quant4/4(dout0_4) -> Delay97/1
  quant4/2(clip_out) -> Delay95/1
  quant4/1(sync_out) -> Delay94/1
  x0_even/1 -> Delay32/1, x0/3(din0)
  x0_odd/1 -> Delay33/1, x0/4(din1)
  freq_band/1 -> [band_in]
  sync/1 -> [sync_in]
  [sync_in] -> x0/1(sync)
  y0_even/1 -> x1/3(din0), Delay16/1
  y0_odd/1 -> x1/4(din1), Delay21/1
  [band_in] -> x1/2(freq_band)
  [sync_in] -> x1/1(sync)
  x1/1(sync_out) -> Terminator/1
  x1_even1/1 -> Delay24/1, x2/3(din0)
  x1_odd1/1 -> Delay25/1, x2/4(din1)
  [band_in] -> x2/2(freq_band)
  [sync_in] -> x2/1(sync)
  x2/1(sync_out) -> Terminator2/1
  y1_even1/1 -> Delay28/1, x3/3(din0)
  y1_odd1/1 -> Delay29/1, x3/4(din1)
  [band_in] -> x3/2(freq_band)
  [sync_in] -> x3/1(sync)
  x3/1(sync_out) -> Terminator1/1
  [band_in] -> x0/2(freq_band)
  x0/2(dout0) -> quant4/2(din0)
  x0/3(dout1) -> quant4/3(din1)
  x0/1(sync_out) -> [eq_sync]
  [eq_sync] -> quant4/1(sync)
  Delay1/1 -> full_even_x0/1
  Delay2/1 -> full_odd_x0/1
  Delay8/1 -> quant_odd_y0/1
  Delay7/1 -> quant_even_y0/1
  Delay6/1 -> clip_out_y0/1
  quant1/6(dout1_4) -> Delay8/1
  quant1/4(dout0_4) -> Delay7/1
  quant1/2(clip_out) -> Delay6/1
  x1/2(dout0) -> quant1/2(din0)
  x1/3(dout1) -> quant1/3(din1)
  [eq_sync] -> quant1/1(sync)
  Delay3/1 -> full_even_y0/1
  Delay4/1 -> full_odd_y0/1
  Delay14/1 -> quant_odd_x1/1
  Delay13/1 -> quant_even_x1/1
  Delay12/1 -> clip_out_x1/1
  quant3/6(dout1_4) -> Delay14/1
  quant3/4(dout0_4) -> Delay13/1
  quant3/2(clip_out) -> Delay12/1
  x2/2(dout0) -> quant3/2(din0)
  x2/3(dout1) -> quant3/3(din1)
  [eq_sync] -> quant3/1(sync)
  Delay9/1 -> full_even_x1/1
  Delay10/1 -> full_odd_x1/1
  Delay19/1 -> quant_odd_y1/1
  Delay18/1 -> quant_even_y1/1
  Delay17/1 -> clip_out_y1/1
  quant6/6(dout1_4) -> Delay19/1
  quant6/4(dout0_4) -> Delay18/1
  quant6/2(clip_out) -> Delay17/1
  x3/2(dout0) -> quant6/2(din0)
  x3/3(dout1) -> quant6/3(din1)
  [eq_sync] -> quant6/1(sync)
  Delay20/1 -> full_even_y1/1
  Delay15/1 -> full_odd_y1/1
  quant6/1(sync_out) -> Terminator3/1
  quant3/1(sync_out) -> Terminator5/1
  quant3/3(dout0) -> Terminator16/1
  quant3/5(dout1) -> Terminator17/1
  quant6/3(dout0) -> Terminator25/1
  quant6/5(dout1) -> Terminator26/1
  quant1/1(sync_out) -> Terminator9/1
  quant1/3(dout0) -> Terminator10/1
  quant1/5(dout1) -> Terminator11/1
  quant4/3(dout0) -> Terminator7/1
  quant4/5(dout1) -> Terminator8/1
  Delay5/1 -> Delay15/1
  Delay11/1 -> Delay20/1
  Delay28/1 -> Delay11/1
  Delay29/1 -> Delay5/1
  Delay23/1 -> Delay10/1
  Delay22/1 -> Delay9/1
  Delay25/1 -> Delay23/1
  Delay24/1 -> Delay22/1
  Delay26/1 -> Delay3/1
  Delay27/1 -> Delay4/1
  Delay16/1 -> Delay26/1
  Delay21/1 -> Delay27/1
  Delay30/1 -> Delay1/1
  Delay31/1 -> Delay2/1
  Delay33/1 -> Delay31/1
  Delay32/1 -> Delay30/1
